simulink model "Simulink"  (R2022b)
settings: Solver=VariableStepAuto  StartTime=0.0  StopTime=t_finish  RelTol=1e-3
values from neighbouring files (symbols this model uses):
  a0 = 5    [Zajecia3Matlab.m]
  a1 = 5    [Zajecia3Matlab.m]
  b = 9    [Zajecia3Matlab.m]
  du = 0    [Zajecia3Matlab.m]
  t0 = 10    [Zajecia3Matlab.m]
  u0 = 20    [Zajecia3Matlab.m]
  x0 = b*u0/a0    (= 36)    [Zajecia3Matlab.m]
settings Model: Creator=huber  LastModifiedBy=huber
settings DataIOCC: ReturnWorkspaceOutputs=off

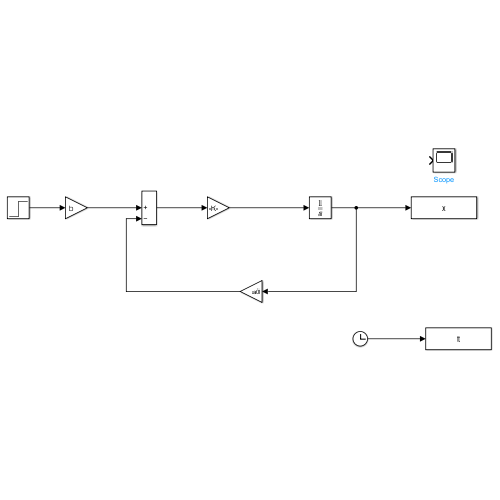
[thumbnail: Simulink's stored preview of the top-level diagram]
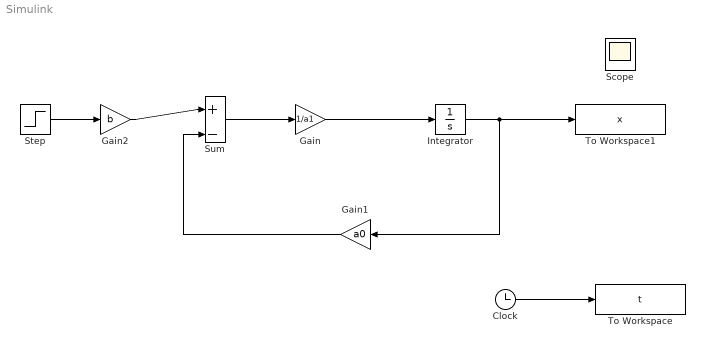
== system Simulink ==
  Clock : Clock
  Gain : Gain  Gain=1/a1
  Gain1 : Gain  Gain=a0
  Gain2 : Gain  Gain=b
  Integrator : Integrator  InitialCondition=x0
  Scope : Scope
  Step : Step  Time=t0  Before=u0  After=u0 + du  SampleTime=0
  Sum : Sum  Inputs=|+-
  To Workspace : ToWorkspace  VariableName=t  SampleTime=-1
  To Workspace1 : ToWorkspace  VariableName=x  SampleTime=-1
  wires:
  Clock/1 -> To Workspace/1
  Gain/1 -> Integrator/1
  Integrator/1 -> Gain1/1, To Workspace1/1
  Sum/1 -> Gain/1
  Step/1 -> Gain2/1
  Gain1/1 -> Sum/2
  Gain2/1 -> Sum/1
